simulink model "sampleModel2083"  (R2023a)
settings: Solver=VariableStepAuto  StartTime=0.0  StopTime=10.0  RelTol=1e-3
libraries: hdlsllib x4, simulink x4
settings Model: Creator=user1  LastModifiedBy=user1

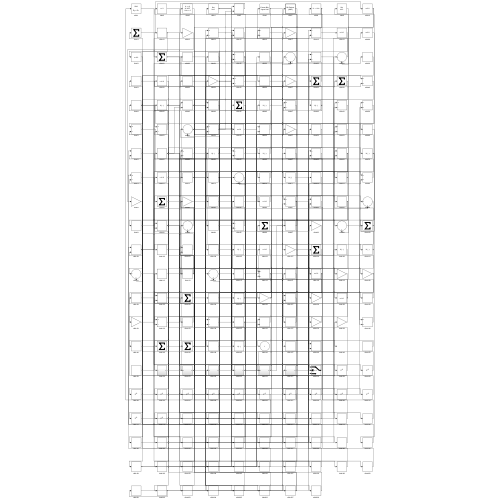
[thumbnail: Simulink's stored preview of the top-level diagram]
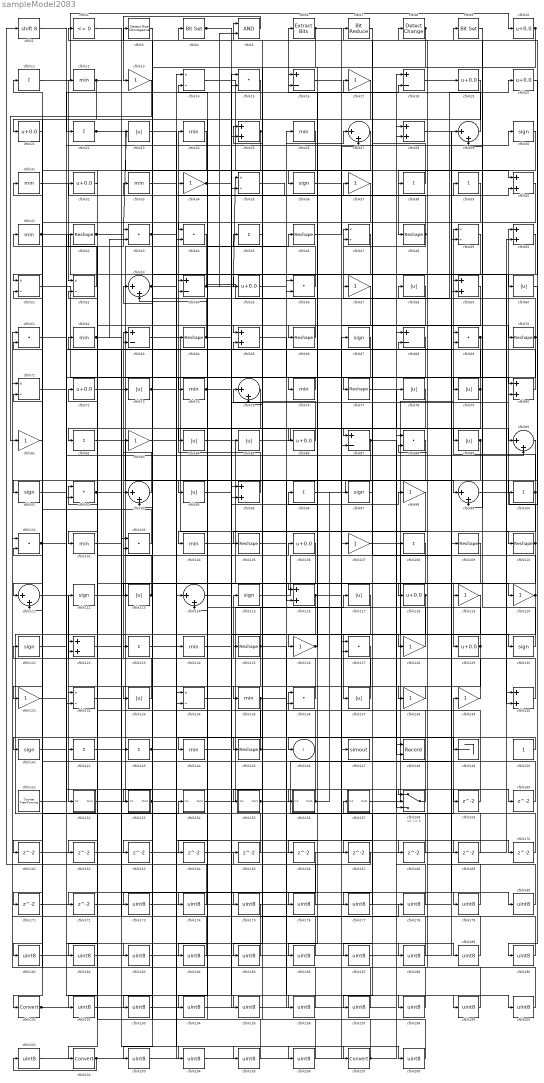
== system sampleModel2083 ==
  cfblk1 : ArithShift  BitShiftNumber=8
  cfblk{10,19..21,32,55,72,86,106,118,129} (11 alike) : Bias  Bias=0.0  SaturateOnIntegerOverflow=off
  cfblk{11,22,38..39,45,82,96,100,108,123,142..143} (12 alike) : Sum  Inputs=+
  cfblk{15,43..44,56,61,69,88,92,101,103,127,136} (12 alike) : DotProduct  OutDataTypeStr=Inherit: Inherit via internal rule
  cfblk{12,24,26,31,33,41,62,74,76,102,104,124,135,144} (14 alike) : MinMax
  cfblk{42,46,48,64,66,70,77,105,109..110,125,145} (12 alike) : Reshape
  cfblk{13,17,34,37,57,81,83,98,107,119..120,126,128,131,138..139} (16 alike) : Gain
  cfblk{27,29,53,75,90,93,99,111,114} (9 alike) : Sum  Inputs=|++
  cfblk{30,36,67,91,97,112,115,121,130,141} (10 alike) : Signum
  cfblk{23,58,60,73,78..79,84..85,89,94,113,117,133,137} (14 alike) : Abs  SaturateOnIntegerOverflow=off
  cfblk{25,28,40,50,59,65,80,95,116,122,140} (11 alike) : Sum
  cfblk{14,35,47,49,51..52,71,132,134} (9 alike) : Product  Inputs=*/  RndMeth=Zero  SaturateOnIntegerOverflow=on
  cfblk147 : ToWorkspace  VariableName=simout  SaveFormat=Timeseries  SampleTime=-1
  cfblk148 : Record  FileSettingsInternal="{\"entries\":[{\"content\":{\"excelSettings\":{\"content\":{},\"type\":\"Streamout.ExcelSettings\"}},\"type\":\"Streamout.FileSettingStorage\",\"uuid\":\"\"}],\"packageUris\":[\"http:\\/\\/schema.mathworks.com\\/mf0\\/streamout_blocks\\/R2020a\"],\"version\":\"1.0\"}"  Layout=[1 1]  SignalsInternal="{\"entries\":[{\"content\":{\"signals\":[{\"content\":{\"blockPath\":[],\"dimensions\":[1],\"domain\":\"\",\"lineColor\":\"#a2142f\",\"plots\":[1],\"port\":1,\"signalID\":6665,\"signalName\":\"XY Graph:1\"},\"type\":\"RecordBlkView.Signal\",\"uuid\":\"\"},{\"content\":{\"blockPath\":[],\"dimensions\":[1],\"domain\":\"\",\"lineColor\":\"#139fff\",\"plots\":[1],\"port\":2,\"signalID\":6668,\"signalName\":\"XY Graph:2\"},\"type\":\"RecordBlkView.Signal\",\"uuid\":\"\"}]},\"type\":\"RecordBlkView.InputSignals\",\"uuid\":\"\"}],\"packageUris\":[\"http:\\/\\/schema.mathworks.com\\/mf0\\/streamout_blocks\\/R2020a\"],\"version\":\"1.0\"}"  VisualizationBindings="{\"xyplotplugin\":{\"info\":[{\"series\":[{\"bindingParametersList\":[{\"parameter\":\"X-Axis\",\"signalID\":6665,\"signalName\":\"XY Graph:1\"},{\"parameter\":\"Y-Axis\",\"signalID\":6668,\"signalName\":\"XY Graph:2\"}],\"seriesID\":59450}],\"subplotID\":1}]}}"  CompatibilityTag=XY  st=-1
  cfblk149 : Terminator
  cfblk150 : Constant  SampleTime=-1
  cfblk151 : hdlsllib/Sources/Counter Free-Running  NumBits=16  tsamp=-1
  cfblk152 : Subsystem
      settings: LibrarySourceBlock=|
      | hdlsllib/Ports &
      | Subsystems/Subsystem
  cfblk153 : Subsystem
      settings: LibrarySourceBlock=|
      | hdlsllib/Ports &
      | Subsystems/Subsystem
  cfblk154 : Subsystem
      settings: LibrarySourceBlock=|
      | hdlsllib/Ports &
      | Subsystems/Subsystem
  cfblk155 : Subsystem
      settings: LibrarySourceBlock=|
      | hdlsllib/Ports &
      | Subsystems/Subsystem
  cfblk156 : Subsystem
      settings: LibrarySourceBlock=|
      | hdlsllib/Ports &
      | Subsystems/Subsystem
  cfblk157 : Subsystem
      settings: LibrarySourceBlock=|
      | hdlsllib/Ports &
      | Subsystems/Subsystem
  cfblk158 : Switch  SaturateOnIntegerOverflow=off  InputSameDT=off
  cfblk{159..172} (14 alike) : Delay  SampleTime=1
  cfblk{16,18,54,63,68,87} (6 alike) : Sum  Inputs=+-
  cfblk{173..190,192..201,203..206,208} (33 alike) : DataTypeConversion  OutDataTypeStr=uint8  SaturateOnIntegerOverflow=off  RndMeth=Floor
  cfblk191 : DataTypeConversion  SaturateOnIntegerOverflow=off  RndMeth=Floor
  cfblk2 : hdlsllib/Logic and Bit Operations/Compare To Zero  relop=<=  OutDataTypeStr=boolean
  cfblk202 : DataTypeConversion  SaturateOnIntegerOverflow=off  RndMeth=Floor
  cfblk207 : DataTypeConversion  SaturateOnIntegerOverflow=off  RndMeth=Floor
  cfblk3 : hdlsllib/Logic and Bit Operations/Detect Rise Nonnegative  vinit=0  OutDataTypeStr=boolean
  cfblk4 : simulink/Logic and Bit Operations/Bit Set  iBit=0
      settings: LibrarySourceBlock=|
      | hdlsllib/Logic and Bit
      | Operations/Bit Set
  cfblk5 : Logic  AllPortsSameDT=off  OutDataTypeStr=boolean
  cfblk6 : simulink/Logic and Bit Operations/Extract Bits  bitsToExtract=Upper half  numBits=8  bitIdxRange=[0 7]  outScalingMode=Preserve fixed-point scaling
      settings: LibrarySourceBlock=|
      | hdlsllib/Logic and Bit
      | Operations/Extract Bits
  cfblk7 : hdlsllib/Logic and Bit Operations/Bit Reduce  mode=AND
  cfblk8 : simulink/Logic and Bit Operations/Detect Change  vinit=0  OutDataTypeStr=boolean
      settings: LibrarySourceBlock=|
      | hdlsllib/Logic and Bit
      | Operations/Detect
      | Change
  cfblk9 : simulink/Logic and Bit Operations/Bit Set  iBit=0
      settings: LibrarySourceBlock=|
      | hdlsllib/Logic and Bit
      | Operations/Bit Set
  cfblk146 : Outport  VectorParamsAs1DForOutWhenUnconnected=off
  wires:
  cfblk100/1 -> cfblk49/1, cfblk140/2
  cfblk95/1 -> cfblk24/1
  cfblk56/1 -> cfblk21/1
  cfblk44/1 -> cfblk20/1
  cfblk99/1 -> cfblk4/1
  cfblk75/1 -> cfblk82/1
  cfblk154/1(Out1) -> cfblk117/1
  cfblk15/1 -> cfblk44/1
  cfblk5/1 -> cfblk13/1
  cfblk119/1 -> cfblk137/1
  cfblk152/1(Out1) -> cfblk46/1
  cfblk63/1 -> cfblk110/1
  cfblk13/1 -> cfblk81/1
  cfblk112/1 -> cfblk106/1
  cfblk89/1 -> cfblk181/1, cfblk194/1
  cfblk21/1 -> cfblk154/1(In1)
  cfblk27/1 -> cfblk44/2
  cfblk77/1 -> cfblk89/1
  cfblk133/1 -> cfblk63/1
  cfblk136/1 -> cfblk115/1
  cfblk22/1 -> cfblk36/1, cfblk38/1
  cfblk11/1 -> cfblk10/1
  cfblk30/1 -> cfblk48/1
  cfblk153/1(Out1) -> cfblk103/2, cfblk170/1
  cfblk137/1 -> cfblk31/1
  cfblk138/1 -> cfblk135/1
  cfblk98/1 -> cfblk145/1
  cfblk111/1 -> cfblk152/1(In1)
  cfblk78/1 -> cfblk132/1
  cfblk157/1(Out1) -> cfblk59/1
  cfblk73/1 -> cfblk206/1, cfblk208/1
  cfblk72/1 -> cfblk54/1
  cfblk113/1 -> cfblk93/1, cfblk52/2
  cfblk35/1 -> cfblk37/1
  cfblk76/1 -> cfblk74/1
  cfblk155/1(Out1) -> cfblk139/1, cfblk59/2
  cfblk24/1 -> cfblk51/1
  cfblk57/1 -> cfblk66/1
  cfblk90/1 -> cfblk91/1
  cfblk104/1 -> cfblk120/1
  cfblk55/1 -> cfblk27/1
  cfblk54/1 -> cfblk35/1, cfblk5/2
  cfblk134/1 -> cfblk98/1
  cfblk36/1 -> cfblk107/1
  cfblk82/1 -> cfblk148/1
  cfblk107/1 -> cfblk130/1
  cfblk93/1 -> cfblk73/1
  cfblk14/1 -> cfblk40/1
  cfblk118/1 -> cfblk132/2, cfblk184/1
  cfblk48/1 -> cfblk12/1, cfblk47/2
  cfblk84/1 -> cfblk147/1
  cfblk38/1 -> cfblk2/1
  cfblk125/1 -> cfblk142/1, cfblk54/2, cfblk158/1, cfblk199/1
  cfblk110/1 -> cfblk50/1, cfblk129/1
  cfblk139/1 -> cfblk112/1
  cfblk19/1 -> cfblk105/1
  cfblk126/1 -> cfblk96/1, cfblk16/1
  cfblk1/1 -> cfblk22/1
  cfblk150/1 -> cfblk146/1
  cfblk42/1 -> cfblk23/1, cfblk158/3
  cfblk4/1 -> cfblk85/1, cfblk168/1
  cfblk81/1 -> cfblk131/1
  cfblk59/1 -> cfblk84/1
  cfblk69/1 -> cfblk75/2, cfblk187/1
  cfblk97/1 -> cfblk7/1
  cfblk31/1 -> cfblk52/1
  cfblk39/1 -> cfblk153/1(In1)
  cfblk51/1 -> cfblk134/2
  cfblk85/1 -> cfblk90/1
  cfblk144/1 -> cfblk69/1
  cfblk156/1(Out1) -> cfblk93/2, cfblk97/1
  cfblk140/1 -> cfblk25/1
  cfblk53/1 -> cfblk14/1, cfblk39/1
  cfblk74/1 -> cfblk80/2, cfblk156/1(In1), cfblk174/1
  cfblk122/1 -> cfblk143/1
  cfblk25/1 -> cfblk65/1, cfblk162/1
  cfblk87/1 -> cfblk119/1, cfblk116/2, cfblk167/1
  cfblk131/1 -> cfblk90/2
  cfblk47/1 -> cfblk104/1
  cfblk65/1 -> cfblk80/1
  cfblk8/1 -> cfblk166/1, cfblk185/1
  cfblk58/1 -> cfblk102/1
  cfblk32/1 -> cfblk122/1
  cfblk43/1 -> cfblk114/1, cfblk86/1
  cfblk116/1 -> cfblk141/1, cfblk148/2
  cfblk17/1 -> cfblk113/1
  cfblk33/1 -> cfblk55/1
  cfblk18/1 -> cfblk19/1
  cfblk6/1 -> cfblk133/1, cfblk70/1
  cfblk26/1 -> cfblk191/1
  cfblk151/1 -> cfblk30/1
  cfblk115/1 -> cfblk49/2
  cfblk80/1 -> cfblk14/2
  cfblk34/1 -> cfblk15/2, cfblk76/1, cfblk94/1
  cfblk158/1 -> cfblk136/1
  cfblk7/1 -> cfblk77/1
  cfblk128/1 -> cfblk75/1
  cfblk12/1 -> cfblk111/1, cfblk176/1
  cfblk23/1 -> cfblk149/1
  cfblk120/1 -> cfblk144/1, cfblk17/1, cfblk203/1
  cfblk103/1 -> cfblk41/1
  cfblk50/1 -> cfblk95/2
  cfblk83/1 -> cfblk207/1
  cfblk41/1 -> cfblk140/1, cfblk158/2
  cfblk101/1 -> cfblk111/2, cfblk64/1, cfblk43/1
  cfblk143/1 -> cfblk69/2, cfblk16/2
  cfblk29/1 -> cfblk6/1
  cfblk86/1 -> cfblk5/1
  cfblk96/1 -> cfblk99/1
  cfblk10/1 -> cfblk99/2, cfblk126/1
  cfblk62/1 -> cfblk118/1, cfblk79/1, cfblk43/2
  cfblk67/1 -> cfblk155/1(In1)
  cfblk79/1 -> cfblk87/1, cfblk42/1
  cfblk20/1 -> cfblk60/1
  cfblk130/1 -> cfblk9/1
  cfblk92/1 -> cfblk116/1, cfblk204/1
  cfblk145/1 -> cfblk92/1, cfblk57/1
  cfblk64/1 -> cfblk32/1, cfblk128/1
  cfblk132/1 -> cfblk65/2
  cfblk66/1 -> cfblk33/1
  cfblk46/1 -> cfblk27/2
  cfblk135/1 -> cfblk40/2, cfblk171/1
  cfblk127/1 -> cfblk202/1
  cfblk105/1 -> cfblk58/1
  cfblk91/1 -> cfblk18/2
  cfblk9/1 -> cfblk29/2
  cfblk129/1 -> cfblk53/2, cfblk62/1, cfblk138/1
  cfblk70/1 -> cfblk47/1, cfblk92/2, cfblk100/1
  cfblk52/1 -> cfblk11/1
  cfblk141/1 -> cfblk159/1
  cfblk159/1 -> cfblk95/1
  cfblk102/1 -> cfblk160/1
  cfblk160/1 -> cfblk51/2
  cfblk40/1 -> cfblk161/1
  cfblk161/1 -> cfblk134/1
  cfblk162/1 -> cfblk50/2
  cfblk49/1 -> cfblk163/1
  cfblk163/1 -> cfblk136/2
  cfblk37/1 -> cfblk164/1
  cfblk164/1 -> cfblk35/2
  cfblk165/1 -> cfblk101/2
  cfblk167/1 -> cfblk1/1
  cfblk168/1 -> cfblk122/2
  cfblk16/1 -> cfblk169/1
  cfblk169/1 -> cfblk63/2
  cfblk170/1 -> cfblk53/1
  cfblk171/1 -> cfblk29/1
  cfblk106/1 -> cfblk172/1
  cfblk172/1 -> cfblk67/1
  cfblk3/1 -> cfblk173/1
  cfblk173/1 -> cfblk78/1
  cfblk174/1 -> cfblk3/1
  cfblk45/1 -> cfblk175/1
  cfblk176/1 -> cfblk45/1
  cfblk88/1 -> cfblk177/1
  cfblk177/1 -> cfblk157/1(In1)
  cfblk175/1 -> cfblk178/1
  cfblk178/1 -> cfblk88/1
  cfblk2/1 -> cfblk179/1
  cfblk179/1 -> cfblk88/2
  cfblk28/1 -> cfblk180/1
  cfblk180/1 -> cfblk8/1
  cfblk181/1 -> cfblk28/1
  cfblk166/1 -> cfblk182/1
  cfblk182/1 -> cfblk28/2
  cfblk71/1 -> cfblk183/1
  cfblk183/1 -> cfblk87/2
  cfblk184/1 -> cfblk71/1
  cfblk185/1 -> cfblk71/2
  cfblk109/1 -> cfblk186/1
  cfblk186/1 -> cfblk34/1
  cfblk187/1 -> cfblk109/1
  cfblk61/1 -> cfblk188/1
  cfblk188/1 -> cfblk103/1
  cfblk114/1 -> cfblk189/1
  cfblk189/1 -> cfblk61/1
  cfblk60/1 -> cfblk190/1
  cfblk190/1 -> cfblk61/2
  cfblk191/1 -> cfblk25/2, cfblk15/1
  cfblk117/1 -> cfblk192/1
  cfblk192/1 -> cfblk26/1
  cfblk108/1 -> cfblk193/1
  cfblk193/1 -> cfblk56/2
  cfblk194/1 -> cfblk108/1
  cfblk121/1 -> cfblk195/1
  cfblk195/1 -> cfblk56/1
  cfblk94/1 -> cfblk196/1
  cfblk196/1 -> cfblk121/1
  cfblk68/1 -> cfblk197/1
  cfblk197/1 -> cfblk165/1
  cfblk142/1 -> cfblk198/1
  cfblk198/1 -> cfblk68/1
  cfblk199/1 -> cfblk68/2
  cfblk124/1 -> cfblk200/1
  cfblk200/1 -> cfblk101/1
  cfblk201/1 -> cfblk124/1
  cfblk202/1 -> cfblk201/1, cfblk18/1
  cfblk203/1 -> cfblk127/1
  cfblk204/1 -> cfblk127/2
  cfblk123/1 -> cfblk205/1
  cfblk205/1 -> cfblk72/1
  cfblk206/1 -> cfblk123/1
  cfblk207/1 -> cfblk125/1, cfblk114/2
  cfblk208/1 -> cfblk83/1

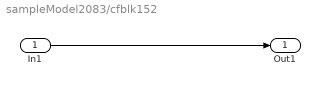
== system sampleModel2083/cfblk152 ==
  In1 : Inport
  Out1 : Outport
  wires:
  In1/1 -> Out1/1

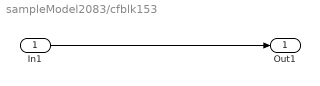
== system sampleModel2083/cfblk153 ==
  In1 : Inport
  Out1 : Outport
  wires:
  In1/1 -> Out1/1

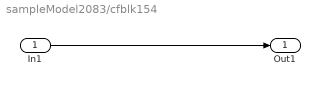
== system sampleModel2083/cfblk154 ==
  In1 : Inport
  Out1 : Outport
  wires:
  In1/1 -> Out1/1

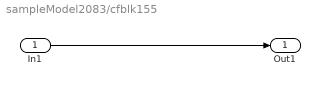
== system sampleModel2083/cfblk155 ==
  In1 : Inport
  Out1 : Outport
  wires:
  In1/1 -> Out1/1

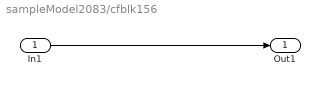
== system sampleModel2083/cfblk156 ==
  In1 : Inport
  Out1 : Outport
  wires:
  In1/1 -> Out1/1

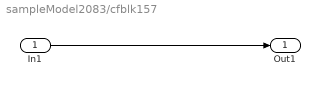
== system sampleModel2083/cfblk157 ==
  In1 : Inport
  Out1 : Outport
  wires:
  In1/1 -> Out1/1
